simulink model "Collision_08_Compare_Forces"  (R2016b)
settings: Solver=ode15s  StartTime=0.0  StopTime=5  MaxStep=1e-3  RelTol=1e-8  AbsTol=1e-8  EnableMultiTasking=on
PostLoadFcn:
  | warning off Simulink:Engine:UsingDefaultMaxStepSize
StartFcn:
  | tic;
StopFcn:
  | Elapsed_Sim_Time = toc;
  | disp(['Elapsed Sim Time = ' num2str(Elapsed_Sim_Time)]);
undefined symbols (not defined in the file): Extr_Data_Ring, X, Y, Z
libraries: sm_lib x39, nesl_utility x6, Contact_Forces_Lib x5
(part 2 of 2)

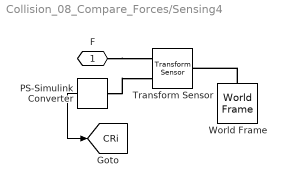
== system Collision_08_Compare_Forces/Sensing4 ==
  PS-Simulink Converter : nesl_utility/PS-Simulink Converter  PhysicalDomain=network_engine_domain  SubClassName=ps_output  LeftPortType=input  RightPortType=output  PseudoPeriodic=off  Frequencies=[]  Unit=1  AffineConversion=off
  Transform Sensor : sm_lib/Frames and Transforms/Transform Sensor  MeasurementFrame=World  SenseAngle=off  SenseAxis=off  SenseAngle1=off  SenseAngle2=off  SenseAngle3=off  SenseQ=off  SenseR=off  SenseOmegaX=off  SenseOmegaY=off  SenseOmegaZ=off  SenseOmega1=off  SenseOmega2=off  SenseOmega3=off  SenseQDot=off  SenseRDot=off  SenseAlphaX=off  SenseAlphaY=off  SenseAlphaZ=off  SenseAlpha1=off  SenseAlpha2=off  SenseAlpha3=off  SenseQDDot=off  SenseRDDot=off  SenseX=off  SenseY=off  SenseZ=on  SenseRad=off  SenseAzim=off  SenseDist=off  SenseInc=off  SenseXDot=off  SenseYDot=off  SenseZDot=off  SenseRadDot=off  SenseAzimDot=off  SenseDistDot=off  SenseIncDot=off  SenseXDDot=off  SenseYDDot=off  SenseZDDot=off  SenseRadDDot=off  SenseAzimDDot=off  SenseDistDDot=off  SenseIncDDot=off
  World Frame : sm_lib/Frames and Transforms/World Frame
  F : PMIOPort  Port=1  Side=Left
  tag scope: CRi=global
  wires:
  PS-Simulink Converter/1 -> [CRi]
  connections:
  PS-Simulink Converter/LConn1 -- Transform Sensor/RConn2
  F/RConn1 -- Transform Sensor/RConn1
  World Frame/RConn1 -- Transform Sensor/LConn1

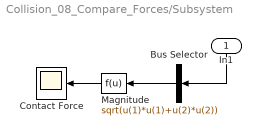
== system Collision_08_Compare_Forces/Subsystem ==
  In1 : Inport
  Bus Selector : BusSelector  OutputSignals=FCir.Fy,FCir.Fx  OutputAsBus=on
  Contact Force : Scope
  Magnitude : Fcn  Expr=sqrt(u(1)*u(1)+u(2)*u(2))
  wires:
  Magnitude/1 -> Contact Force/1
  In1/1 -> Bus Selector/1
  Bus Selector/1 -> Magnitude/1

== system Collision_08_Compare_Forces/Subsystem1 ==
  In1 : Inport
  Bus Selector : BusSelector  OutputSignals=Normal Force
  Contact Force : Scope
  wires:
  In1/1 -> Bus Selector/1
  Bus Selector/1 -> Contact Force/1  "<Normal Force>"

== system Collision_08_Compare_Forces/Subsystem2 ==
  In1 : Inport
  Bus Selector : BusSelector  OutputSignals=Normal Force
  Contact Force : Scope
  wires:
  In1/1 -> Bus Selector/1
  Bus Selector/1 -> Contact Force/1  "<Normal Force>"

== system Collision_08_Compare_Forces/Subsystem3 ==
  In1 : Inport
  Bus Selector : BusSelector  OutputSignals=Normal Force  OutputAsBus=on
  Contact Force : Scope
  wires:
  In1/1 -> Bus Selector/1
  Bus Selector/1 -> Contact Force/1

== system Collision_08_Compare_Forces/Subsystem4 ==
  In1 : Inport
  Bus Selector : BusSelector  OutputSignals=Normal Force
  Contact Force : Scope
  wires:
  In1/1 -> Bus Selector/1
  Bus Selector/1 -> Contact Force/1  "<Normal Force>"
